simulink model "DCmotor06"  (R2019b)
settings: Solver=ode45  StartTime=0.0  StopTime=1  MaxStep=1e-6  RelTol=1e-3
undefined symbols (not defined in the file): TN
libraries: powerlib x8, simulink x1
Description:
  | 简单的不可逆，开环，无制动通道
settings Model: Creator=DELL  LastModifiedBy=Inspiron
settings DataIOCC: ReturnWorkspaceOutputs=off
settings DebuggingCC: ArithmeticOperatorsInVariantConditions=warning
settings SFSimCC: SimUseLocalCustomCode=off  CustomCodeUndefinedFunction=UseInterfaceOnly
settings RTWCC: RTWUseLocalCustomCode=off
settings CodeAppCC: StateflowObjectComments=on
settings SimscapeCC: SimscapeNormalizeSystem=off

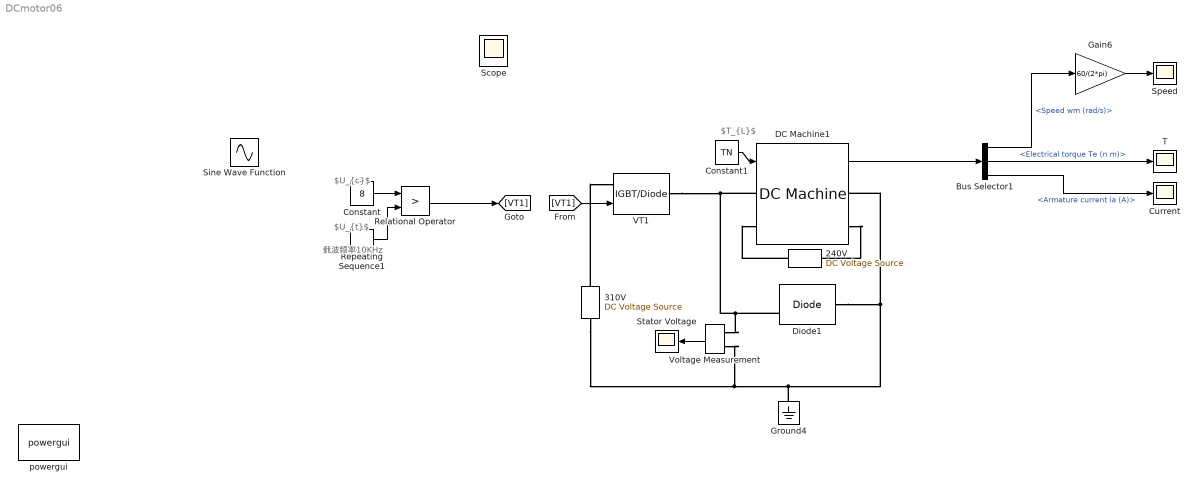
== system DCmotor06 ==
  note: 载波频率10KHz
  note: $U_{t}$
  note: $U_{c}$
  note: $T_{L}$
  240V : powerlib/Electrical Sources/DC Voltage Source  Amplitude=240  Measurements=None
      settings: SourceProductName=Simscape Electrical
  310V : powerlib/Electrical Sources/DC Voltage Source  Amplitude=310  Measurements=None
      settings: SourceProductName=Simscape Electrical
  Bus Selector1 : BusSelector  OutputSignals=Speed wm (rad/s),Electrical torque Te (n m),Armature current ia (A)
  Constant : Constant  Value=8
  Constant1 : Constant  Value=TN
  Current : Scope
  DC Machine1 : powerlib/Machines/DC Machine  PresetModel=No  MechanicalLoad=Torque TL  FieldType=Wound  ShowDetailedParameters=on  MeasurementBus=off  RLa="[ 0.6  0.012]"  RLf="[ 240  120]"  Laf=1.8  MachineConstant=Torque constant (N.m/A)  Ke=1.8  Kt=1.8  J=0.05  Bm=0  Tf=0  w0=0  Ifinit=1  TsPowergui=0  TsBlock=-1
      settings: SourceProductName=Simscape Electrical
  Diode1 : powerlib/Power Electronics/Diode  Ron=0.001  Lon=0  Vf=0.8  IC=0  UseSnubber=0  Rs=500  Cs=250e-9  Measurements=on
      settings: SourceProductName=Simscape Electrical
  Gain6 : Gain  Gain=60/(2*pi)
  Ground4 : powerlib/Elements/Ground  LConnTagsString=a
      settings: SourceProductName=Simscape Electrical
  Relational Operator : RelationalOperator  Operator=>  OutDataTypeStr=boolean  RndMeth=Simplest
  Repeating Sequence1 : simulink/Sources/Repeating Sequence  rep_seq_t=[0 1e-4 ]  rep_seq_y=[0 10]
  Scope : Scope  NumInputPorts=3
  Sine Wave Function : Sin  Amplitude=5  Bias=5  Frequency=2*pi*1000  SampleTime=0
  Speed : Scope
  Stator Voltage : Scope
  T : Scope
  VT1 : powerlib/Power Electronics/IGBT//Diode  Ron=1e-3  Rs=1e5  Cs=inf  Measurements=off
      settings: SourceProductName=Simscape Electrical
  Voltage Measurement : powerlib/Measurements/Voltage Measurement  PhasorSimulation=off  OutputType=Complex  PSBequivalent=0
      settings: SourceProductName=Simscape Electrical
  powergui : powerlib/powergui  Priority=1  SimulationMode=Continuous  SampleTime=50e-6  frequency=60  Iterations=50  frequencyindice=0  Pbase=100e6  ErrMax=1e-4  UnitsV=kV  UnitsW=MW  buscounter=0  FunctionMessages=off  echomessages=off  EnableUseOfTLC=off  CurrentSourceSwitches=on  DisableSnubberDevices=off  DisableRonSwitches=off  DisableVfSwitches=off  DisplayEquations=off  AutomaticDiscreteSolvers=off  SolverType=Tustin/Backward Euler (TBE)  Interpol=off  ExternalGateDelay=off  methode=off  Ts=10  x0status=blocks  SPID=off  SwTol=0  HookPort=off  NonlinearTolerance=1e-4  nMaxIteration=100  ContinueOnMaxIteration=off  RestoreLinks=warning  ResistiveCurrentMeasurement=off  Frange=[0:2:500]  Ylog=off  Xlog=on  ShowGrid=off  save=off  variable=ZData  structure=0  ZoomFFT=off  StartTime=0.0  cycles=1  DisplayStyle=1  fundamental=60  FreqAxis=off  MaxFrequency=1000  frequencyindicesteady=1  RmsSteady=1  display=off
      settings: SourceProductName=Simscape Electrical
  wires:
  Bus Selector1/3 -> Current/1  "<Armature current ia (A)>"
  DC Machine1/1 -> Bus Selector1/1
  Gain6/1 -> Speed/1
  Voltage Measurement/1 -> Stator Voltage/1
  Bus Selector1/1 -> Gain6/1  "<Speed wm (rad/s)>"
  [VT1] -> VT1/1
  Constant1/1 -> DC Machine1/1
  Bus Selector1/2 -> T/1  "<Electrical torque Te (n m)>"
  Repeating Sequence1/1 -> Relational Operator/2
  Relational Operator/1 -> [VT1]
  Constant/1 -> Relational Operator/1
  connections:
  310V/RConn1 -- VT1/LConn1
  DC Machine1/LConn1 -- Voltage Measurement/LConn1 -- Diode1/RConn1 -- VT1/RConn1
  Ground4/LConn1 -- Voltage Measurement/LConn2 -- 310V/LConn1 -- Diode1/LConn1 -- DC Machine1/RConn1
  DC Machine1/RConn2 -- 240V/LConn1
  240V/RConn1 -- DC Machine1/LConn2
